simulink model "snizovac_novy"  (Simulink 7.6)
settings: Solver=ode1  StartTime=0.0  StopTime=0.15  FixedStep=1e-07  RelTol=1e-3
undefined symbols (not defined in the file): plecsedit
libraries: simulink x1
settings Model: Creator=dragounj  LastModifiedBy=kaskaj

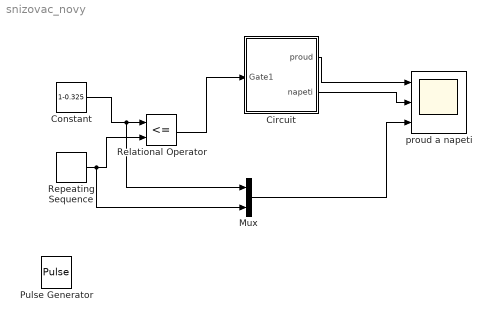
== system snizovac_novy ==
  Circuit : Subsystem  LoadFcn=plecsedit('sl', 200);  InitFcn=plecsedit('sl', 214);  StartFcn=plecsedit('sl', 208);  StopFcn=plecsedit('sl', 209);  mask(PlecsCircuit){}
      mask init:
      | % PLACE CUSTOM INITIALIZATIONS ABOVE
      | % DO NOT REMOVE
      | plecsedit('sl', 215);
      | % DO NOT REMOVE
      settings: CopyFcn=plecsedit('sl', 203);  DeleteFcn=plecsedit('sl', 205);  UndoDeleteFcn=plecsedit('sl', 206);  PreSaveFcn=plecsedit('sl', 211);  PostSaveFcn=plecsedit('sl', 201);  NameChangeFcn=plecsedit('sl', 210);  DestroyFcn=plecsedit('sl', 207);  PreCopyFcn=plecsedit('sl', 216);  OpenFcn=plecsedit('sl', 202);  ErrorFcn=plerrorfcn
      mask Display: disp('PLECS\nCircuit')
  Constant : Constant  Value=1-0.325
  Mux : Mux  Inputs=2
  Pulse Generator : DiscretePulseGenerator  PulseType=Time based  Period=0.005  PulseWidth=60
  Relational Operator : RelationalOperator  Operator=<=  OutDataTypeStr=boolean
  Repeating Sequence : simulink/Sources/Repeating Sequence  SystemSampleTime=-1  rep_seq_t=[0 0.5 1]/1000  rep_seq_y=[0 1 0]
  proud a napeti : Scope  NumInputPorts=3
      settings: TimeRange=0.01  YMin=70~0~0  YMax=160~200~1
  wires:
  Circuit/1(proud) -> proud a napeti/1
  Circuit/2(napeti) -> proud a napeti/2
  Constant/1 -> Relational Operator/1, Mux/1
  Repeating Sequence/1 -> Relational Operator/2, Mux/2
  Relational Operator/1 -> Circuit/1(Gate1)
  Mux/1 -> proud a napeti/3

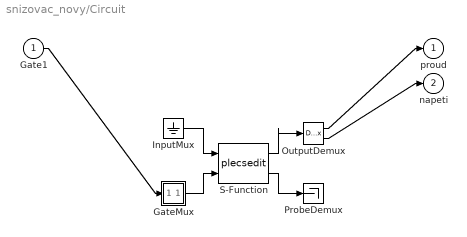
== system snizovac_novy/Circuit ==
  Gate1 : Inport
  " GateMux " : Subsystem
      mask Display: disp('Mux')
  " InputMux " : Ground
  " OutputDemux " : Demux  Outputs=[ 1 1 ]
  " ProbeDemux " : Terminator
  " S-Function " : S-Function  FunctionName=plecsedit  EnableBusSupport=off
  proud : Outport
  napeti : Outport  Port=2
  wires:
  " S-Function "/1 -> " OutputDemux "/1
  " InputMux "/1 -> " S-Function "/1
  " GateMux "/1(Out) -> " S-Function "/2
  " S-Function "/2 -> " ProbeDemux "/1
  Gate1/1 -> " GateMux "/1(In1)
  " OutputDemux "/1 -> proud/1
  " OutputDemux "/2 -> napeti/1

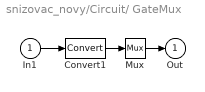
== system snizovac_novy/Circuit/ GateMux  ==
  In1 : Inport
  Convert1 : DataTypeConversion  SaturateOnIntegerOverflow=on  RndMeth=Zero
  Mux : Mux  Inputs=[ 1 ]
  Out : Outport
  wires:
  Mux/1 -> Out/1
  In1/1 -> Convert1/1
  Convert1/1 -> Mux/1
